simulink library "xpclib"  (Simulink 6.0)
settings: Solver=ode45  SolverMode=SingleTasking  StartTime=0.0  StopTime=10.0  RelTol=1e-3
values from neighbouring files (symbols this model uses):
  base = get_param( gcb, 'base' )    [maddiamondmm.m]    (also in maddiamondmm32frame.m; maddsmm16at.m; mdadsmm16at.m; mdiortddm64x0.m = hex2dec(addr(3:end)))
  block = find_system(bdroot,                          'FollowLinks', 'on',                          'LookUnderMasks', 'all',                          'MaskType', type )    [mdionipci6527.m]
  count = count + 1    (= 5)    [mdecodestate.m]
  port = get_param( gcb, 'port' )    [mdionipci6527.m]    (also in mdiortddm64x0.m = get_param(blocks{i}, 'port'))
undefined symbols (not defined in the file or in its folder): CIO, devid, DIO24, genixlib, get, handlers, irq, mbaseserialmask, mbwaudpmc, mdacbpcidas, mdiamondemeraldmask, mgenix, mmodemcontrol, mquamask, mrs232, msc150checks, mtargetboxleds, mtargetboxwatchdog, mxpccan, PCI, sizeof, vendid
libraries: xpclib x384, simulink x6
(part 3 of 7)

== system xpclib/RS232/Diamond ==
  "Emerald-MM " : Subsystem  PropExecContextAcrossSSBoundary=on
  "Emerald-MM8 " : Subsystem  PropExecContextAcrossSSBoundary=on

== system xpclib/RS232/Mainboard ==
  Baseboard Serial : Subsystem  InitFcn=mbaseserialmask(4,2);  TreatAsAtomicUnit=on  PropExecContextAcrossSSBoundary=on  mask(Baseboard RS232 Send Receive){group=Board Setup, port=1, irqnum=4, saddr1=0x3f8, saddr2=0x3e8, config=Com1/Com3, baud1=115200, parity1=None, ndata1=8, nstop1=1, fifomode1=16 deep, rlevel1=half full, automode1=on, xmtfifosize1=1024, xmtdatatype1=8 bit uint null terminated, rcvfifosize1=1024, rcvmaxread1=1024, rcvminread1=1, rcvusedelim1=on, rcvdelim1=13, rcvdatatype1=count+16 bit uint, rcvsampletime1=-1, baud2=115200, parity2=None, ndata2=8, nstop2=1, fifomode2=16 deep, rlevel2=half full, automode2=off, xmtfifosize2=1024, xmtdatatype2=8 bit uint null terminated, rcvfifosize2=1024, rcvmaxread2=1024, rcvminread2=1, rcvusedelim2=on, rcvdelim2=13, rcvdatatype2=count+16 bit uint, rcvsampletime2=-1}
      mask prompts: group "Parameter group:"; port "Port to modify:"; irqnum "IRQ number:"; saddr1 "First port address:"; saddr2 "Second port address:"; config "Configuration:"; baud1 "Baud rate:"; parity1 "Parity:"; ndata1 "Data bits:"; nstop1 "Stop bits:"; fifomode1 "Hardware fifo size:"; rlevel1 "Receive fifo interrupt level:"; automode1 "Auto RTS/CTS:"; xmtfifosize1 "Transmit software fifo size:"; xmtdatatype1 "Transmit fifo data type:"; rcvfifosize1 "Receive software fifo size:"; rcvmaxread1 "Receive maximum read:"; rcvminread1 "Receive minimum read:"; rcvusedelim1 "Read to delimiter:"; rcvdelim1 "Delimiter:"; rcvdatatype1 "Receive data type:"; rcvsampletime1 "Receive SampleTime:"; baud2 "Baud rate:"; parity2 "Parity:"; ndata2 "Data bits:"; nstop2 "Stop bits:"; fifomode2 "Hardware fifo size:"; rlevel2 "Receive fifo interrupt level:"; automode2 "Auto RTS/CTS:"; xmtfifosize2 "Transmit software fifo size:"; xmtdatatype2 "Transmit fifo data type:"; rcvfifosize2 "Receive software fifo size:"; rcvmaxread2 "Receive maximum read:"; rcvminread2 "Receive minimum read:"; rcvusedelim2 "Read to delimiter:"; rcvdelim2 "Delimiter:"; rcvdatatype2 "Receive data type:"; rcvsampletime2 "Receive SampleTime:"
      mask help:
      | Baseboard
      | RS232 Send Receive Subsystem
      mask init:
      | [addr1, addr2, maskdisplay] = mbaseserialmask( 1, 2 );
      | baddr1 = addr1;
      | baddr2 = addr2;
      | mbaseserialmask( 3, 2 );
      | set_param( gcb, 'MaskDisplay', maskdisplay );
      mask Help: helpview(fullfile(docroot, 'mapfiles', 'xpc.map'), 'Baseboard_Serial_Subsystem')
      mask StyleString: popup(Board Setup|Basic Setup|Transmit Setup|Receive Setup),popup(1|2),edit,edit,edit,popup(Com1/none|Com2/none|Com1/Com3|Com2/Com4|none/Com3|none/Com4|Custom),popup(921600|460800|230400|115200|57600|38400|19200|9600|4800|2400|1200|600|300|110),popup(None|Even|Odd|Mark|Space),popup(5|6|7|8),popup(1|2),popup(64 deep|16 deep|1 deep),popup(1|quarter full|half full|almost full),checkbox,edit,popup(count+32 bit int|count+32 bit uint|count+16 bit int|count+16 bit uint|8 bit int null terminated|8 bit uint null terminated),edit,edit,edit,checkbox,edit,popup(count+32 bit int|count+32 bit uint|count+16 bit int|count+16 bit uint|8 bit int null terminated|8 bit uint null terminated),edit,popup(921600|460800|230400|115200|57600|38400|19200|9600|4800|2400|1200|600|300|110),popup(None|Even|Odd|Mark|Space),popup(5|6|7|8),popup(1|2),popup(64 deep|16 deep|1 deep),popup(1|quarter full|half full|almost full),checkbox,edit,popup(count+32 bit int|count+32 bit uint|count+16 bit int|count+16 bit uint|8 bit int null terminated|8 bit uint null terminated),edit,edit,edit,checkbox,edit,popup(count+32 bit int|count+32 bit uint|count+16 bit int|count+16 bit uint|8 bit int null terminated|8 bit uint null terminated),edit
      mask CallbackString:
      | mbaseserialmask( 2, 2 );
      | |mbaseserialmask( 2, 2 );||||mbaseserialmask( 2, 2 );
      | ||||||||||||||||||||||||||||||||
      mask Display: disp('Baseboard\nRS232\nSend Receive')port_label('input',1,'XMT1');port_label('input',2,'XMT3');port_label('output',1,'RCV1');port_label('output',2,'RCV3');
  Baseboard Serial Internal  blocks : Subsystem  PropExecContextAcrossSSBoundary=on
  Modem Control : S-Function  InitFcn=mmodemcontrol(4)  FunctionName=modemcontrolbase  Parameters=addr, boardtype, rts, dtr, count  mask(Baseboard Modem Control){rts=on, dtr=on, config=Com1, addr=0x3f8}
      mask prompts: config "Configuration:"; addr "Base address:"
      mask help:
      | Baseboard
      | Modem Control
      mask init:
      | count = 0;
      | boardtype = 4;
      | [maskdisplay, count, addr] = mmodemcontrol( 2, rts, dtr, boardtype, config, addr );
      | addr = hex2dec( addr(3:end) );
      | set_param( gcb, 'MaskDisplay', maskdisplay );
      mask Help: helpview(fullfile(docroot, 'mapfiles', 'xpc.map'), 'Baseboard_MODEM_Control')
      mask StyleString: checkbox,checkbox,popup(Com1|Com2|Com3|Com4|Custom),edit
      mask CallbackString:
      | ||mmodemcontrol( 1 );
      | |
      mask Display: disp('Baseboard\nModem Control');port_label('input',1,'RTS');port_label('input',2,'DTR');
  Modem Status : S-Function  FunctionName=modemstatusbase  Parameters=addr, boardtype, cts, dsr, ring, dcd, count, sampletime  mask(Modem Status){cts=on, dsr=on, ring=on, dcd=on, sampletime=-1, config=Com1, addr=0x3f8}
      mask prompts: ring "RI:"; config "Configuration:"; addr "Base address:"
      mask help:
      | Baseboard
      | Modem Status
      mask init:
      | count = 0;
      | boardtype = 4;
      | [maskdisplay, count, addr] = mmodemstatus( 2, cts, dsr, ring, dcd, boardtype, config, addr );
      | addr = hex2dec( addr(3:end) );
      | set_param( gcb, 'MaskDisplay', maskdisplay );
      mask Help: helpview(fullfile(docroot, 'mapfiles', 'xpc.map'), 'Baseboard_MODEM_Status')
      mask StyleString: checkbox,checkbox,checkbox,checkbox,edit,popup(Com1|Com2|Com3|Com4|Custom),edit
      mask CallbackString:
      | |||||mmodemstatus( 1 );
      | |
      mask Display: disp('Baseboard\nModem Status');port_label('output',1,'CTS');port_label('output',2,'DSR');port_label('output',3,'RI');port_label('output',4,'DCD');

== system xpclib/RS232/Quatech ==
  ESC-100 : Subsystem  PropExecContextAcrossSSBoundary=on
  QSC-100 : Subsystem  PropExecContextAcrossSSBoundary=on
  QSC-200/300 : Subsystem  PropExecContextAcrossSSBoundary=on

== system xpclib/RS232/Setup  ==
  S-Function : S-Function  FunctionName=rs232_setup  Parameters=port,baudrate,databit, stopbit, parity, protocol, sendbuf, recbuf, 0

== system xpclib/RS232/Synchronous Mode ==
  note: V1.0 compatible
  "RS232 " : S-Function  FunctionName=rs232sendrec  Parameters=port, inStr, outStr, inport, outport, numinports, numoutports, formatsendinfo, formatrecinfo, waitarg, dtypes, ts, numeom, timeoutarg  mask(rs232sendrec){port=COM1, blockvar=[], ts=0.1}
      mask prompts: blockvar "Message struct name:"; ts "Sample time:"
      mask help:
      | RS-232
      | Mainboard
      | Send/Receive
      mask init:
      | inStr = '';
      | outStr = '';
      | [inStr,outStr,dtypes,maskdisplay,maskdescription,inport,outport, numinports, numoutports, formatsendinfo, formatrecinfo, waitarg, numeom, timeoutarg] = mrs232 (1, blockvar, 3);
      | set_param(gcb,'MaskDisplay',maskdisplay);
      | set_param(gcb,'MaskDescription',maskdescription);
      mask Help: helpview(fullfile(docroot, 'mapfiles', 'xpc.map'), 'RS232_Synchronous-Mode_RS232')
      mask StyleString: popup(COM1|COM2|COM3|COM4),edit,edit
      mask Display: disp('RS-232\nMainboard\nSend/Receive');
  "Send & Receive " : Subsystem  PropExecContextAcrossSSBoundary=on  mask(rs232sendrec){port=COM2, formatsend='start,%f,stop;', formatrec='start,%f,stop;', numb=1, ts=0.01}
      mask prompts: formatsend "Send format:"; formatrec "Receive format:"; numb "Number of end-of-message characters:"; ts "Sample time:"
      mask Help: helpview(fullfile(docroot, 'mapfiles', 'xpc.map'), 'RS232_Synchronous-Mode_Send-&-Receive')
      mask StyleString: popup(COM1|COM2|COM3|COM4),edit,edit,edit,edit
      mask Display: disp('RS232\nMainboard\nSend/Receive');

== system xpclib/Shared Memory/SBS Broadcast Memory ==
  "SBS25x0 init " : S-Function  FunctionName=memsbs25x0init  Parameters=get(node,'BT_REG_CTRL_ARG'),get(node,'BT_REG_MEM_ARG'),get(node,'WIT'),[],pci  mask(SBS 25x0 Initialization){node=[], pci=-1}
      mask prompts: node "Node struct:"; pci "PCI slot (-1: autosearch)"
      mask help: Configures 5565 shared-memory board produced by VMIC Inc. This is a required block for any model that uses shared memory with the VMIC 5565. It configures important registers on the board according to the user-defined node structure.
      mask init:
      | node=smnodesbs25x0(node);
      mask Help: helpview(fullfile(docroot, 'mapfiles', 'xpc.map'),'SBS_25x0_Init')
      mask Display: disp('init')
  "SBS25x0 read " : S-Function  FunctionName=memsbs25x0read  Parameters=base(partition(1)), sizeof(partition(1)),ts, pci, errport  mask(SBS 25x0 Read){partition=[], ts=0.001, pci=-1, errport=off}
      mask prompts: partition "Partition struct:"; ts "Sampletime:"; pci "PCI slot (-1: autosearch)"; errport "Error Status Port"
      mask help: Reads blocks of data (32-bit words) from shared memory. Should be combined with '5565 unpack' to define data partitioning.
      mask init:
      | partition=smpartsbs25x0(partition);
      mask Help: helpview(fullfile(docroot, 'mapfiles', 'xpc.map'),'SBS_25x0_Read')
      mask Display:
      | disp('read')
      | port_label('output',1,'ud')
  "SBS25x0 write " : S-Function  FunctionName=memsbs25x0write  Parameters=base(partition(1)), sizeof(partition(1)),ts, pci, errport  mask(SBS 25x0 Write){partition=[], ts=0.001, pci=-1, errport=off}
      mask prompts: partition "Partition struct:"; ts "Sampletime:"; pci "PCI slot (-1: autosearch)"; errport "Error Status Port"
      mask help: Writes blocks of data (32-bit words) to shared-memory. Should be combined with '5565 pack' to define data partitioning.
      mask init:
      | partition=smpartsbs25x0(partition);
      mask Help: helpview(fullfile(docroot, 'mapfiles', 'xpc.map'),'SBS_25x0_Write')
      mask Display: disp('write')

== system xpclib/Shared Memory/Systran ==
  Change endianess : xpclib/Shared Memory/Change endianess  numInp=1  lengthIn=Byte
  "SC150 init " : S-Function  InitFcn=msc150checks(1)  FunctionName=memscramnetinit  Parameters=node.Interface.Internal.CSRs, node.Interface.Internal.ACRAMinfo, pci  mask(SC150 Init){node=[], pci=-1}
      mask prompts: node "Node struct:"; pci "PCI slot (-1: autosearch)"
      mask help:
      | SC150
      | Systran
      | Initialization
      mask init:
      | node=completenodestruct(node);
      mask Help: helpview(fullfile(docroot, 'mapfiles', 'xpc.map'),'Systran_SC150_Init')
      mask Display: disp('init')
  "SC150 pack " : xpclib/Shared Memory/Shared Memory Pack   partition=[]
  "SC150 read " : S-Function  FunctionName=memscramnetread  Parameters=partition(1).Internal.Address, partition(1).Internal.NDwords, ts, pci  mask(SC150 Read){partition=[], ts=0.001, pci=-1}
      mask prompts: partition "Partition struct:"; ts "Sampletime:"; pci "PCI slot (-1: autosearch)"
      mask help:
      | SC150
      | Systran
      | Read
      mask init:
      | partition=completepartitionstruct(partition);
      mask Help: helpview(fullfile(docroot, 'mapfiles', 'xpc.map'),'Systran_SC150_Read')
      mask Display: disp('read')
  SC150 rearm : S-Function  FunctionName=memscramnetrearm  Parameters=partition.Internal.Address, partition.Internal.NDwords, ts, pci  mask(SC150 Rearm){partition=[], ts=0.001, pci=-1}
      mask prompts: partition "Partition struct:"; ts "Sampletime:"; pci "PCI slot (-1: autosearch)"
      mask help:
      | SC150
      | Systran
      | Rearm
      mask init:
      | partition=completepartitionstruct(partition);
      mask Help: helpview(fullfile(docroot, 'mapfiles', 'xpc.map'),'Systran_SC150_Rearm')
      mask Display: disp('rearm')
  "SC150 unpack " : xpclib/Shared Memory/Shared Memory Unpack   partition=[]
  "SC150 write " : S-Function  FunctionName=memscramnetwrite  Parameters=partition(1).Internal.Address, partition(1).Internal.NDwords, ts, pci  mask(SC150 Write){partition=[], ts=0.001, pci=-1}
      mask prompts: partition "Partition struct:"; ts "Sampletime:"; pci "PCI slot (-1: autosearch)"
      mask help:
      | SC150
      | Systran
      | Write
      mask init:
      | partition=completepartitionstruct(partition);
      mask Help: helpview(fullfile(docroot, 'mapfiles', 'xpc.map'),'Systran_SC150_Write')
      mask Display: disp('write')

== system xpclib/Shared Memory/VMIC ==
  5565 broadcast : S-Function  FunctionName=mem5565netbroadcast  Parameters=ninterrupt,target, ts, pci  mask(5565 Network Interrupts){target=-1, ninterrupt=1, ts=0.001, pci=-1}
      mask prompts: target "Target Node (-1 : Global)"; ninterrupt "Interrupt Number"; ts "Sampletime:"; pci "PCI slot (-1: autosearch)"
      mask help: Generates network interrupts at the specified sample rate.
      mask Help: helpview(fullfile(docroot, 'mapfiles', 'xpc.map'),'VMIC_5565_Broadcast')
      mask StyleString: edit,popup(1|2|3|Initialization),edit,edit
      mask Display:
      | disp('Broadcast')
      | port_label('Input',1,'En')
      | port_label('Input',2,'Data')
  "5565 init " : S-Function  FunctionName=mem5565netinit  Parameters=node.Interface.Internal.LCSR1, node.Interface.Internal.LIER,node.Interface.Internal.INodeID,pci  mask(5565 Initialization){node=[], pci=-1}
      mask prompts: node "Node struct:"; pci "PCI slot (-1: autosearch)"
      mask help: Configures 5565 shared-memory board produced by VMIC Inc. This is a required block for any model that uses shared memory with the VMIC 5565. It configures important registers on the board according to the user-defined node structure.
      mask init:
      | node=completenodestruct(node,'5565');
      mask Help: helpview(fullfile(docroot, 'mapfiles', 'xpc.map'),'VMIC_5565_Init')
      mask Display: disp('init')
  "5565 pack " : xpclib/Shared Memory/Shared Memory Pack   partition=[]
  "5565 read " : S-Function  FunctionName=mem5565netread  Parameters=partition(1).Internal.Address, partition(1).Internal.NDwords, ts, pci, errport  mask(5565 Memory Read){partition=[], ts=0.001, pci=-1, errport=off}
      mask prompts: partition "Partition struct:"; ts "Sampletime:"; pci "PCI slot (-1: autosearch)"; errport "Error Status Port"
      mask help: Reads blocks of data (32-bit words) from shared memory. Should be combined with '5565 unpack' to define data partitioning.
      mask init:
      | partition=completepartitionstruct(partition);
      mask Help: helpview(fullfile(docroot, 'mapfiles', 'xpc.map'),'VMIC_5565_Read')
      mask Display:
      | disp('read')
      | port_label('output',1,'ud')
  "5565 unpack  " : xpclib/Shared Memory/Shared Memory Unpack   partition=[]
  "5565 write " : S-Function  FunctionName=mem5565netwrite  Parameters=partition(1).Internal.Address, partition(1).Internal.NDwords, ts, pci, errport  mask(5565 Write){partition=[], ts=0.001, pci=-1, errport=off}
      mask prompts: partition "Partition struct:"; ts "Sampletime:"; pci "PCI slot (-1: autosearch)"; errport "Error Status Port"
      mask help: Writes blocks of data (32-bit words) to shared-memory. Should be combined with '5565 pack' to define data partitioning.
      mask init:
      | partition=completepartitionstruct(partition);
      mask Help: helpview(fullfile(docroot, 'mapfiles', 'xpc.map'),'VMIC_5565_Write')
      mask Display: disp('write')
  Change endianess : xpclib/Shared Memory/Change endianess  numInp=1  lengthIn=Byte

== system xpclib/Signal Conditioning/add2 ==
  "CIO-DIO24 " : S-Function  AncestorBlock=genixlib/CIO-DIO24  LoadFcn=mgenix(1)  InitFcn=mgenix(1)  FunctionName=genixisa8255  Parameters=initData, offset8255, baseAddress, control8255  mask(genixisa8255){fileName=, baseaddress=0x300}
      mask prompts: fileName "Genix initialization file (path\file):"; baseaddress "Base address (i.e. 0xd000):"
      mask help:
      | CIO-DIO24
      | ComputerBoards
      | Genix
      mask init:
      | baseAddress=hex2dec(baseaddress(3:end));
      | boardType=1;
      | control8255=0;
      | offset8255=0;
      | initData=[];
      | [initData, offset8255, control8255]=mgenix(2, fileName, baseAddress, 1);
      mask Help: helpview(fullfile(docroot, 'mapfiles', 'xpc.map'), 'add2_CIO-DIO24_SignalConditioning')
      mask Display: disp('CIO-DIO24\nComputerBoards\nGenix');
  "PCI-DIO24 " : S-Function  AncestorBlock=genixlib/PCI-DIO24  LoadFcn=mgenix(1)  InitFcn=mgenix(1)  FunctionName=genixpci8255  Parameters=initData, offset8255, pciSlot, control8255  mask(genixpci8255){fileName=, pciSlot=-1}
      mask prompts: fileName "Genix initialization file (path\file):"; pciSlot "PCI slot (-1: autosearch):"
      mask help:
      | PCI-DIO24
      | ComputerBoards
      | Genix
      mask init:
      | boardType=1;
      | control8255=0;
      | offset8255=0;
      | initData=[];
      | [initData, offset8255, control8255]=mgenix(2, fileName, pciSlot, 2);
      mask Help: helpview(fullfile(docroot, 'mapfiles', 'xpc.map'), 'add2_PCI-DIO24_SignalConditioning')
      mask Display: disp('PCI-DIO24\nComputerBoards\nGenix');

== system xpclib/Synchro Resolver/NAII ==

== system xpclib/Synchro Resolver/SBS  Technologies ==

== system xpclib/Thermo couple/Measurement Computing ==

== system xpclib/Watchdog/Acces IO ==
  "WDG-CSM " : S-Function  FunctionName=wdaciowdgcsm  Parameters=wdtime,showreset,sampletime,baseaddress  mask(wdaciowdgcsm){wdtime=1, showreset=off, sampletime=0.001, baseaddress=0x300}
      mask prompts: wdtime "Watchdog time [s] (20us-4800s):"; showreset "Show reset port"; sampletime "Sample time:"; baseaddress "Base address (i.e. 0xd000):"
      mask help:
      | WDG-CSM
      | ACCES I/O
      | Watchdog
      mask init:
      | baseaddress=hex2dec(baseaddress(3:end));
      mask Help: helpview(fullfile(docroot, 'mapfiles', 'xpc.map'), 'AccesIO_WDG-CSM_Watchdog')
      mask Display: disp('WDG-CSM\nACCES I/O\nWatchdog');

== system xpclib/Watchdog/MathWorks ==
  Watchdog : S-Function  InitFcn=mtargetboxwatchdog(1);  FunctionName=targetboxwatchdog  Parameters=units, interval, portReset, kybdReset, mouseReset, reboot, sampleTime  mask(targetboxwatchdog){units=seconds, interval=255, portReset=on, kybdReset=off, mouseReset=off, reboot=off, sampleTime=0.001}
      mask prompts: units "Timeout units:"; interval "Timeout interval (1-255):"; portReset "Show reset port (R)"; kybdReset "Reset upon keyboard activity"; mouseReset "Reset upon mouse activity"; reboot "Reboot upon expiration of watchdog"; sampleTime "Sample time:"
      mask help:
      | TargetBox 10x120x
      | The MathWorks
      | Watchdog
      mask init:
      | phase = 2;
      | [maskDisplay, maskDescription] = mtargetboxwatchdog( phase, interval, portReset, sampleTime );
      | set_param(gcb,'MaskDescription',maskDescription);
      | set_param(gcb,'MaskDisplay',maskDisplay);
      mask Help: helpview(fullfile(docroot, 'mapfiles', 'xpc_targetbox.map'), 'TheMathWorks_TargetBox10x120x_Watchdog')
      mask StyleString: popup(seconds|minutes),edit,checkbox,checkbox,checkbox,checkbox,edit
      mask Display: disp('TargetBox 10x120x\nThe MathWorks\nWatchdog');port_label('input', 1, 'R');

== system xpclib/Watchdog/Versalogic ==

== system xpclib/CAN/Softing/CAN-AC2-104 SJA 1000 ==
  FIFO Mode : Subsystem  PropExecContextAcrossSSBoundary=on
  "Receive " : S-Function  FunctionName=canac2104receive  Parameters=canPort, ids, ididx, output, ts, board  mask(canac2104receive){board=1, canPort=CAN 1, range=Standard (11-bit), ids=[0], output=Data, inten=off, ts=0.001, ididx=[0]}
      mask prompts: canPort "CAN port:"; range "CAN identifier range:"; ids "Identifiers:"; output "Output port options:"; inten "Generate interrupts"; ts "Sample time:"
      mask help:
      | Softing
      | CAN-AC2-104
      | with SJA1000
      mask init:
      | mxpccanicon('CAN-AC2-104','Receive',canPort,range,ids,board)
      mask Help: helpview(fullfile(docroot, 'mapfiles', 'xpc.map'), 'Softing_CAN-AC2-104-SJA-1000_Receive')
      mask StyleString: popup(1|2|3),popup(CAN 1|CAN 2),popup(Standard (11-bit)|Extended (29-bit)),edit,popup(Data|Data - Status|Data - Timestamp|Data - Status - Timestamp),checkbox,edit,edit
      mask Display: text(0.05,0.75,'CAN-AC2-104 B1','horizontalAlignment','left');text(0.05,0.5,'CAN 1 - Receive','horizontalAlignment','left');text(0.05,0.25,'Standard 11bit','horizontalAlignment','left');port_label('output',1,'0');
  "Send " : S-Function  FunctionName=canac2104send  Parameters=canPort, ids, ididx, output, ts, sizesout, board  mask(canac2104send){board=1, canPort=CAN 1, range=Standard (11-bit), ids=[0], sizes=[8], output=off, ts=0.001, ididx=[0]}
      mask prompts: canPort "CAN port:"; range "CAN identifier range:"; ids "Identifiers:"; sizes "Data frame sizes:"; output "Show status output ports"; ts "Sample time:"
      mask help:
      | Softing
      | CAN-AC2-104
      | with SJA1000
      mask init:
      | if isempty(sizes), sizesout=8; end;
      | if length(sizes)==1, sizesout=sizes*ones(1,length(ids)); else, sizesout=sizes; end;
      | if length(sizesout)~=length(ids), error('Identifier vector and Data Frame Size Vector must have the same length');end
      | if ~isempty(find(sizesout<1|sizesout>8)), error('Data Frame Sizes must be in the range 1..8'); end;
      | mxpccanicon('CAN-AC2-104','Send',canPort,range,ids,board)
      mask Help: helpview(fullfile(docroot, 'mapfiles', 'xpc.map'), 'Softing_CAN-AC2-104-SJA-1000_Send')
      mask StyleString: popup(1|2|3),popup(CAN 1|CAN 2),popup(Standard (11-bit)|Extended (29-bit)),edit,edit,checkbox,edit,edit
      mask Display: text(0.98,0.75,'CAN-AC2-104 B1','horizontalAlignment','right');text(0.98,0.5,'CAN 1 - Send','horizontalAlignment','right');text(0.98,0.25,'Standard 11bit','horizontalAlignment','right');port_label('input',1,'0');
  "Setup " : S-Function  InitFcn=mxpccan(1);  FunctionName=canac2104setup  Parameters=can1UserBR, can2UserBR, can1SendS, can1RecS, can2SendS, can2RecS, can1SendE, can1RecE, can2SendE, can2RecE, can1RecSI, can1RecEI, can2RecSI, can2RecEI, initarray, termarray, ioBaseAddress, memBaseAddress, intNo, board  mask(canac2104setup){board=1, can1Baudrate=1 MBaud, can1UserBR=[1,1,4,3], can2Baudrate=1 MBaud, can2UserBR=[1,1,4,3], init=[], term=[], ioBaseAddressL=0x300, memBaseAddressL=0xd0000, intNo=None}
      mask prompts: can1Baudrate "CAN 1 - baud rate:"; can1UserBR "CAN 1 - user defined baud rate:"; can2Baudrate "CAN 2 - baud rate:"; can2UserBR "CAN 2 - user defined baud rate:"; init "Initialization command structure:"; term "Termination:"; ioBaseAddressL "I/O base address:"; memBaseAddressL "Memory base address:"; intNo "Interrupt line:"
      mask help:
      | Softing
      | CAN-AC2-104
      | with SJA1000
      mask init:
      | initarray=0;
      | termarray=0;
      | ioBaseAddress=768;
      | memBaseAddress=819200;
      | if strcmp(intNo,'None'), intNo='0'; end
      | intNo=str2num(intNo);
      | [can1UserBR, can2UserBR, can1SendS, can1SendE, can2SendS, can2SendE, can1RecS, can1RecE, can2RecS, can2RecE, can1RecSI, can1RecEI, can2RecSI, can2RecEI, initarray, termarray, ioBaseAddress, memBaseAddress]= mxpccan(2, 1, can1Baudrate, can1UserBR, can2Baudrate, can2UserBR, init, term, ioBaseAddressL, memBaseAddressL, board);
      mask Help: helpview(fullfile(docroot, 'mapfiles', 'xpc.map'), 'Softing_CAN-AC2-104-SJA-1000_Setup')
      mask StyleString: popup(1|2|3),popup(1 MBaud|800 kBaud|500 kBaud|250 kBaud|125 kBaud|100 kBaud|10 kBaud|User defined),edit,popup(1 MBaud|800 kBaud|500 kBaud|250 kBaud|125 kBaud|100 kBaud|10 kBaud|User defined),edit,edit,edit,edit,edit,popup(None|5|9|10|11|12|15)
      mask Display: disp(['CAN-AC2-104 B',num2str(board),'\nCAN 1 / CAN 2\nStandard / Extended'])

== system xpclib/CAN/Softing/CAN-AC2-ISA Intel 527 ==
  "Receive " : S-Function  FunctionName=canac2isaereceive  Parameters=canPort, ids, ididx, output, ts, board  mask(canac2isaereceive){board=1, canPort=CAN 1, range=Standard (11-bit), ids=[0], output=Data, inten=off, ts=0.001, ididx=[0]}
      mask prompts: canPort "CAN port:"; range "CAN identifier range:"; ids "Identifiers:"; output "Output port options:"; inten "Generate interrupts"; ts "Sample time:"
      mask help:
      | Softing
      | CAN-AC2-ISA
      | with Intel 82527
      mask init:
      | board=0;
      | mxpccanicon('CAN-AC2-ISA','Receive',canPort,range,ids,board)
      mask Help: helpview(fullfile(docroot, 'mapfiles', 'xpc.map'), 'Softing_CAN-AC2-ISA-Intel-527_Receive')
      mask StyleString: popup(1|2|3),popup(CAN 1|CAN 2),popup(Standard (11-bit)|Extended (29-bit)),edit,popup(Data|Data - Status|Data - Timestamp|Data - Status - Timestamp),checkbox,edit,edit
      mask Display: text(0.05,0.75,'CAN-AC2-ISA','horizontalAlignment','left');text(0.05,0.5,'CAN 1 - Receive','horizontalAlignment','left');text(0.05,0.25,'Standard 11bit','horizontalAlignment','left');port_label('output',1,'0');
  "Send " : S-Function  FunctionName=canac2isaesend  Parameters=canPort, ids, ididx, output, ts, sizesout, board  mask(canac2isaesend){board=1, canPort=CAN 1, range=Standard (11-bit), ids=[0], sizes=[8], output=off, ts=0.001, ididx=[0]}
      mask prompts: canPort "CAN port:"; range "CAN identifier range:"; ids "Identifiers:"; sizes "Data frame sizes:"; output "Show status output ports"; ts "Sample time:"
      mask help:
      | Softing
      | CAN-AC2-ISA
      | with Intel 82527
      mask init:
      | if isempty(sizes), sizesout=8; end;
      | if length(sizes)==1, sizesout=sizes*ones(1,length(ids)); else, sizesout=sizes; end;
      | if length(sizesout)~=length(ids), error('Identifier vector and Data Frame Size Vector must have the same length');end
      | if ~isempty(find(sizesout<1|sizesout>8)), error('Data Frame Sizes must be in the range 1..8'); end;
      | board=0;
      | mxpccanicon('CAN-AC2-ISA','Send',canPort,range,ids,board)
      mask Help: helpview(fullfile(docroot, 'mapfiles', 'xpc.map'), 'Softing_CAN-AC2-ISA-Intel-527_Send')
      mask StyleString: popup(1|2|3),popup(CAN 1|CAN 2),popup(Standard (11-bit)|Extended (29-bit)),edit,edit,checkbox,edit,edit
      mask Display: text(0.98,0.75,'CAN-AC2-ISA','horizontalAlignment','right');text(0.98,0.5,'CAN 1 - Send','horizontalAlignment','right');text(0.98,0.25,'Standard 11bit','horizontalAlignment','right');port_label('input',1,'0');
  "Setup " : S-Function  InitFcn=mxpccan(1);  FunctionName=canac2isaesetup  Parameters=can1UserBR, can2UserBR, can1SendS, can1RecS, can2SendS, can2RecS, can1SendE, can1RecE, can2SendE, can2RecE, can1RecSI, can1RecEI, can2RecSI, can2RecEI, initarray, termarray, ioBaseAddress, memBaseAddress, intNo, board  mask(canac2isaesetup){board=1, can1Baudrate=1 MBaud, can1UserBR=[1,1,4,3], can2Baudrate=1 MBaud, can2UserBR=[1,1,4,3], init=[], term=[], memBaseAddressL=2 (16k): D4000-D7FFF}
      mask prompts: can1Baudrate "CAN 1 - baud rate:"; can1UserBR "CAN 1 - user defined baud rate:"; can2Baudrate "CAN 2 - baud rate:"; can2UserBR "CAN 2 - user defined baud rate:"; init "Initialization command structure:"; term "Termination:"; memBaseAddressL "Memory base address (i.e. 0xd000):"
      mask help:
      | Softing
      | CAN-AC2-ISA
      | with Intel 82527
      mask init:
      | board=1;
      | initarray=0;
      | termarray=0;
      | ioBaseAddress=768;
      | ioBaseAddressL='0x300';
      | memBaseAddress=819200;
      | intNo='None';
      | if strcmp(intNo,'None'), intNo='0'; end
      | intNo=str2num(intNo);
      | [can1UserBR, can2UserBR, can1SendS, can1SendE, can2SendS, can2SendE, can1RecS, can1RecE, can2RecS, can2RecE, can1RecSI, can1RecEI, can2RecSI, can2RecEI, initarray, termarray, ioBaseAddress, memBaseAddress]= mxpccan(2, 4, can1Baudrate, can1UserBR, can2Baudrate, can2UserBR, init, term, ioBaseAddressL, memBaseAddressL, board);
      | ioBaseAddress=768;
      | memBaseAddress=memBaseAddressL;
      mask Help: helpview(fullfile(docroot, 'mapfiles', 'xpc.map'), 'Softing_CAN-AC2-ISA-Intel-527_Setup')
      mask StyleString: popup(1),popup(1 MBaud|800 kBaud|500 kBaud|250 kBaud|125 kBaud|100 kBaud|10 kBaud|User defined),edit,popup(1 MBaud|800 kBaud|500 kBaud|250 kBaud|125 kBaud|100 kBaud|10 kBaud|User defined),edit,edit,edit,popup(0 (64k): D0000-DFFFF|1 (16k): D0000-D3FFF|2 (16k): D4000-D7FFF|3 (16k): D8000-D8FFF|4 (16k): DC000-DFFFF|5 (16k): E0000-E3FFF|6 (16k): E4000-E7FFF|7 (64k): E0000-EFFFF)
      mask Display: disp(['CAN-AC2-ISA E','\nCAN 1 / CAN 2\nStandard / Extended'])

== system xpclib/CAN/Softing/CAN-AC2-ISA Philips C200 ==
  "Receive " : S-Function  FunctionName=canac2isareceive  Parameters=canPort, ids, ididx, output, ts, board  mask(canac2isareceive){board=1, canPort=CAN 1, range=Standard (11-bit), ids=[0], output=Data, inten=off, ts=0.001, ididx=[0]}
      mask prompts: canPort "CAN port:"; range "CAN identifier range:"; ids "Identifiers:"; output "Output port options:"; inten "Generate interrupts"; ts "Sample time:"
      mask help:
      | Softing
      | CAN-AC2-ISA
      | with Philips PCA 82C200
      mask init:
      | board=0;
      | mxpccanicon('CAN-AC2-ISA','Receive',canPort,range,ids,board)
      mask Help: helpview(fullfile(docroot, 'mapfiles', 'xpc.map'), 'Softing_CAN-AC2-ISA-Philips-C200_Receive')
      mask StyleString: popup(1|2|3),popup(CAN 1|CAN 2),popup(Standard (11-bit)|Extended (29-bit)),edit,popup(Data|Data - Status|Data - Timestamp|Data - Status - Timestamp),checkbox,edit,edit
      mask Display: text(0.05,0.75,'CAN-AC2-ISA','horizontalAlignment','left');text(0.05,0.5,'CAN 1 - Receive','horizontalAlignment','left');text(0.05,0.25,'Standard 11bit','horizontalAlignment','left');port_label('output',1,'0');
  "Send " : S-Function  FunctionName=canac2isasend  Parameters=canPort, ids, ididx, output, ts, sizesout, board  mask(canac2isasend){board=1, canPort=CAN 1, range=Standard (11-bit), ids=[0], sizes=[8], output=off, ts=0.001, ididx=[0]}
      mask prompts: canPort "CAN port:"; range "CAN identifier range:"; ids "Identifiers:"; sizes "Data frame sizes:"; output "Show status output ports"; ts "Sample time:"
      mask help:
      | Softing
      | CAN-AC2-ISA
      | with Philips PCA 82C200
      mask init: same as xpclib/CAN/Softing/CAN-AC2-ISA Intel 527/Send 
      mask Help: helpview(fullfile(docroot, 'mapfiles', 'xpc.map'), 'Softing_CAN-AC2-ISA-Philips-C200_Send')
      mask StyleString: popup(1|2|3),popup(CAN 1|CAN 2),popup(Standard (11-bit)|Extended (29-bit)),edit,edit,checkbox,edit,edit
      mask Display: text(0.98,0.75,'CAN-AC2-ISA','horizontalAlignment','right');text(0.98,0.5,'CAN 1 - Send','horizontalAlignment','right');text(0.98,0.25,'Standard 11bit','horizontalAlignment','right');port_label('input',1,'0');
  "Setup " : S-Function  InitFcn=mxpccan(1);  FunctionName=canac2isasetup  Parameters=can1UserBR, can2UserBR, can1SendS, can1RecS, can2SendS, can2RecS, can1SendE, can1RecE, can2SendE, can2RecE, can1RecSI, can1RecEI, can2RecSI, can2RecEI, initarray, termarray, ioBaseAddress, memBaseAddress, intNo, board  mask(canac2isasetup){board=1, can1Baudrate=1 MBaud, can1UserBR=[1,1,4,3], can2Baudrate=1 MBaud, can2UserBR=[1,1,4,3], init=[], term=[], memBaseAddressL=2 (16k): D4000-D7FFF}
      mask prompts: can1Baudrate "CAN 1 - baud rate:"; can1UserBR "CAN 1 - user defined baud rate:"; can2Baudrate "CAN 2 - baud rate:"; can2UserBR "CAN 2 - user defined baud rate:"; init "Initialization command structure:"; term "Termination:"; memBaseAddressL "Memory base address (i.e. 0xd000):"
      mask help:
      | Softing
      | CAN-AC2-ISA
      | with Philips PCA 82C200
      mask init:
      | board=1;
      | initarray=0;
      | termarray=0;
      | ioBaseAddress=768;
      | ioBaseAddressL='0x300';
      | memBaseAddress=819200;
      | intNo='None';
      | if strcmp(intNo,'None'), intNo='0'; end
      | intNo=str2num(intNo);
      | [can1UserBR, can2UserBR, can1SendS, can1SendE, can2SendS, can2SendE, can1RecS, can1RecE, can2RecS, can2RecE, can1RecSI, can1RecEI, can2RecSI, can2RecEI, initarray, termarray, ioBaseAddress, memBaseAddress]= mxpccan(2, 3, can1Baudrate, can1UserBR, can2Baudrate, can2UserBR, init, term, ioBaseAddressL, memBaseAddressL, board);
      | ioBaseAddress=768;
      | memBaseAddress=memBaseAddressL;
      mask Help: helpview(fullfile(docroot, 'mapfiles', 'xpc.map'), 'Softing_CAN-AC2-ISA-Philips-C200_Setup')
      mask StyleString: popup(1),popup(1 MBaud|800 kBaud|500 kBaud|250 kBaud|125 kBaud|100 kBaud|10 kBaud|User defined),edit,popup(1 MBaud|800 kBaud|500 kBaud|250 kBaud|125 kBaud|100 kBaud|10 kBaud|User defined),edit,edit,edit,popup(0 (64k): D0000-DFFFF|1 (16k): D0000-D3FFF|2 (16k): D4000-D7FFF|3 (16k): D8000-D8FFF|4 (16k): DC000-DFFFF|5 (16k): E0000-E3FFF|6 (16k): E4000-E7FFF|7 (64k): E0000-EFFFF)
      mask Display: disp(['CAN-AC2-ISA ','\nCAN 1 / CAN 2\nStandard'])

== system xpclib/CAN/Softing/CAN-AC2-PCI SJA 1000 ==
  FIFO Mode : Subsystem  PropExecContextAcrossSSBoundary=on
  "Receive " : S-Function  FunctionName=canac2pcireceive  Parameters=canPort, ids, ididx, output, ts, board  mask(canac2pcireceive){board=1, canPort=CAN 1, range=Standard (11-bit), ids=[0], output=Data, inten=off, ts=0.001, ididx=[0]}
      mask prompts: canPort "CAN port:"; range "CAN identifier range:"; ids "Identifiers:"; output "Output port options:"; inten "Generate interrupts"; ts "Sample time:"
      mask help:
      | Softing
      | CAN-AC2-PCI
      | with SJA1000
      mask init:
      | mxpccanicon('CAN-AC2-PCI','Receive',canPort,range,ids,board)
      mask Help: helpview(fullfile(docroot, 'mapfiles', 'xpc.map'), 'Softing_CAN-AC2-PCI-SJA-1000_Receive')
      mask StyleString: popup(1|2|3),popup(CAN 1|CAN 2),popup(Standard (11-bit)|Extended (29-bit)),edit,popup(Data|Data - Status|Data - Timestamp|Data - Status - Timestamp),checkbox,edit,edit
      mask Display: text(0.05,0.75,'CAN-AC2-PCI B1','horizontalAlignment','left');text(0.05,0.5,'CAN 1 - Receive','horizontalAlignment','left');text(0.05,0.25,'Standard 11bit','horizontalAlignment','left');port_label('output',1,'0');
  "Send " : S-Function  FunctionName=canac2pcisend  Parameters=canPort, ids, ididx, output, ts, sizesout, board  mask(canac2pcisend){board=1, canPort=CAN 1, range=Standard (11-bit), ids=[0], sizes=[8], output=off, ts=0.001, ididx=[0]}
      mask prompts: canPort "CAN port:"; range "CAN identifier range:"; ids "Identifiers:"; sizes "Data frame sizes:"; output "Show status output ports"; ts "Sample time:"
      mask help:
      | Softing
      | CAN-AC2-PCI
      | with SJA1000
      mask init:
      | if isempty(sizes), sizesout=8; end;
      | if length(sizes)==1, sizesout=sizes*ones(1,length(ids)); else, sizesout=sizes; end;
      | if length(sizesout)~=length(ids), error('Identifier vector and Data Frame Size Vector must have the same length');end
      | if ~isempty(find(sizesout<1|sizesout>8)), error('Data Frame Sizes must be in the range 1..8'); end;
      | mxpccanicon('CAN-AC2-PCI','Send',canPort,range,ids,board)
      mask Help: helpview(fullfile(docroot, 'mapfiles', 'xpc.map'), 'Softing_CAN-AC2-PCI-SJA-1000_Send')
      mask StyleString: popup(1|2|3),popup(CAN 1|CAN 2),popup(Standard (11-bit)|Extended (29-bit)),edit,edit,checkbox,edit,edit
      mask Display: text(0.98,0.75,'CAN-AC2-PCI B1','horizontalAlignment','right');text(0.98,0.5,'CAN 1 - Send','horizontalAlignment','right');text(0.98,0.25,'Standard 11bit','horizontalAlignment','right');port_label('input',1,'0');
  "Setup " : S-Function  InitFcn=mxpccan(1);  FunctionName=canac2pcisetup  Parameters=can1UserBR, can2UserBR, can1SendS, can1RecS, can2SendS, can2RecS, can1SendE, can1RecE, can2SendE, can2RecE, can1RecSI, can1RecEI, can2RecSI, can2RecEI, initarray, termarray, ioBaseAddress, memBaseAddress, intNo, board, can1bus, can2bus  mask(canac2pcisetup){board=1, can1bus=Highspeed (ISO 11898), can1Baudrate=1 MBaud, can1UserBR=[1,1,4,3], can2bus=Highspeed (ISO 11898), can2Baudrate=1 MBaud, can2UserBR=[1,1,4,3], init=[], term=[], ioBaseAddress=-1}
      mask prompts: can1bus "CAN 1 - physical bus:"; can1Baudrate "CAN 1 - baud rate:"; can1UserBR "CAN 1 - user defined baud rate:"; can2bus "CAN 2 - physical bus:"; can2Baudrate "CAN 2 - baud rate:"; can2UserBR "CAN 2 - user defined baud rate:"; init "Initialization command structure:"; term "Termination:"; ioBaseAddress "PCI slot (-1: autosearch):"
      mask help:
      | Softing
      | CAN-AC2-PCI
      | with SJA1000
      mask init:
      | can1str='';can2str='';
      | if can1bus==2, can1str=' LS'; end;if can2bus==2, can2str=' LS'; end;
      | initarray=0;
      | termarray=0;
      | ioBaseAddressL='0'; memBaseAddressL='0';
      | memBaseAddress=819200;
      | intNo=0;
      | [can1UserBR, can2UserBR, can1SendS, can1SendE, can2SendS, can2SendE, can1RecS, can1RecE, can2RecS, can2RecE, can1RecSI, can1RecEI, can2RecSI, can2RecEI, initarray, termarray]= mxpccan(2, 2, can1Baudrate, can1UserBR, can2Baudrate, can2UserBR, init, term, ioBaseAddressL, memBaseAddressL, board);
      mask Help: helpview(fullfile(docroot, 'mapfiles', 'xpc.map'), 'Softing_CAN-AC2-PCI-SJA-1000_Setup')
      mask StyleString: popup(1|2|3),popup(Highspeed (ISO 11898) |Lowspeed (requires LS module)),popup(1 MBaud|800 kBaud|500 kBaud|250 kBaud|125 kBaud|100 kBaud|10 kBaud|User defined),edit,popup(Highspeed (ISO 11898) |Lowspeed (requires LS module)),popup(1 MBaud|800 kBaud|500 kBaud|250 kBaud|125 kBaud|100 kBaud|10 kBaud|User defined),edit,edit,edit,edit
      mask Display: disp(['CAN-AC2-PCI B',num2str(board),'\nCAN 1',can1str,' / CAN 2',can2str,'\nStandard / Extended'])

== system xpclib/CAN/Utilities/CAN Timeout Detection ==
  u : Inport  LatchInput=off
  Fcn : Fcn  Expr=u>timeout
  Gain1 : Gain  Gain=-1  SaturateOnIntegerOverflow=on
  Memory : Memory  InheritSampleTime=on
  Probe : Probe  ProbeWidth=off  ProbeComplexSignal=off  ProbeSignalDimensions=on
  Relational Operator : RelationalOperator  Operator===  InputSameDT=on
  Sum : Sum  SaturateOnIntegerOverflow=on  InputSameDT=on
  Switch : Switch  Orientation=left  Threshold=0.5  InputSameDT=on
  Terminator : Terminator
  Unit Delay : UnitDelay  Orientation=left  SampleTime=-1
  y : Outport
  wires:
  Memory/1 -> Relational Operator/2
  Unit Delay/1 -> Sum/2
  Switch/1 -> Unit Delay/1
  Gain1/1 -> Switch/3
  Relational Operator/1 -> Switch/2
  Sum/1 -> Switch/1, Fcn/1
  Probe/1 -> Sum/1, Gain1/1
  u/1 -> Memory/1, Probe/1, Relational Operator/1
  Fcn/1 -> y/1
  Probe/2 -> Terminator/1

== system xpclib/Misc./To xPC Target /Subsystem ==
  In1 : Inport  LatchInput=off
  Enable : EnablePort
  S-Function : S-Function  FunctionName=dng2xpc  Parameters=paramid
  wires:
  In1/1 -> S-Function/1

== system xpclib/RS232/Asynchronous Mode/Receive  ==
  S-Function : S-Function  FunctionName=rs232_rec  Parameters=port,formatrec,numb,ts
  Out1 : Outport
  wires:
  S-Function/1 -> Out1/1

== system xpclib/RS232/Asynchronous Mode/Send  ==
  In1 : Inport  LatchInput=off
  S-Function : S-Function  FunctionName=rs232_send  Parameters=port,formatsend,wait,ts
  wires:
  In1/1 -> S-Function/1

== system xpclib/RS232/Diamond/Emerald-MM  ==
  Diamond Emerald-MM : Subsystem  PropExecContextAcrossSSBoundary=on
  Diamond Emerald-MM Serial : Subsystem  InitFcn=mdiamondemeraldmask(4,4);  TreatAsAtomicUnit=on  PropExecContextAcrossSSBoundary=on  mask(Emerald-MM RS232 Send Receive){group=Board Setup, port=1, irqnum=7, saddr1=0x240, baud1=115200, parity1=None, ndata1=8, nstop1=1, fifomode1=16 deep, rlevel1=half full, automode1=on, xmtfifosize1=1024, xmtdatatype1=8 bit uint null terminated, rcvfifosize1=1024, rcvmaxread1=1024, rcvminread1=1, rcvusedelim1=on, rcvdelim1=13, rcvdatatype1=count+16 bit uint, rcvsampletime1=-1, baud2=115200, parity2=None, ndata2=8, nstop2=1, fifomode2=16 deep, rlevel2=half full, automode2=on, xmtfifosize2=1024, xmtdatatype2=8 bit uint null terminated, rcvfifosize2=1024, rcvmaxread2=1024, rcvminread2=1, rcvusedelim2=on, rcvdelim2=13, rcvdatatype2=count+16 bit uint, rcvsampletime2=-1, baud3=115200, parity3=None, ndata3=8, nstop3=1, fifomode3=16 deep, rlevel3=half full, automode3=on, xmtfifosize3=1024, xmtdatatype3=8 bit uint null terminated, rcvfifosize3=1024, rcvmaxread3=1024, rcvminread3=1, rcvusedelim3=on, rcvdelim3=13, rcvdatatype3=count+16 bit uint, rcvsampletime3=-1, baud4=115200, parity4=None, ndata4=8, nstop4=1, fifomode4=16 deep, rlevel4=half full, automode4=on, xmtfifosize4=1024, xmtdatatype4=8 bit uint null terminated, rcvfifosize4=1024, rcvmaxread4=1024, rcvminread4=1, rcvusedelim4=on, rcvdelim4=13, rcvdatatype4=count+16 bit uint, rcvsampletime4=-1}
      mask prompts: group "Parameter group:"; port "Port to modify:"; irqnum "IRQ number:"; saddr1 "First port address:"; baud1 "Baud rate:"; parity1 "Parity:"; ndata1 "Data bits:"; nstop1 "Stop bits:"; fifomode1 "Hardware fifo size:"; rlevel1 "Receive fifo interrupt level:"; automode1 "Auto RTS/CTS:"; xmtfifosize1 "Transmit software fifo size:"; xmtdatatype1 "Transmit fifo data type:"; rcvfifosize1 "Receive software fifo size:"; rcvmaxread1 "Receive maximum read:"; rcvminread1 "Receive minimum read:"; rcvusedelim1 "Read to delimiter:"; rcvdelim1 "Delimiter:"; rcvdatatype1 "Receive data type:"; rcvsampletime1 "Receive SampleTime:"; baud2 "Baud rate:"; parity2 "Parity:"; ndata2 "Data bits:"; nstop2 "Stop bits:"; fifomode2 "Hardware fifo size:"; rlevel2 "Receive fifo interrupt level:"; automode2 "Auto RTS/CTS:"; xmtfifosize2 "Transmit software fifo size:"; xmtdatatype2 "Transmit fifo data type:"; rcvfifosize2 "Receive software fifo size:"; rcvmaxread2 "Receive maximum read:"; rcvminread2 "Receive minimum read:"; rcvusedelim2 "Read to delimiter:"; rcvdelim2 "Delimiter:"; rcvdatatype2 "Receive data type:"; rcvsampletime2 "Receive SampleTime:"; baud3 "Baud rate:"; parity3 "Parity:"; ndata3 "Data bits:"; nstop3 "Stop bits:"; fifomode3 "Hardware fifo size:"; rlevel3 "Receive fifo interrupt level:"; automode3 "Auto RTS/CTS:"; xmtfifosize3 "Transmit software fifo size:"; xmtdatatype3 "Transmit fifo data type:"; rcvfifosize3 "Receive software fifo size:"; rcvmaxread3 "Receive maximum read:"; rcvminread3 "Receive minimum read:"; rcvusedelim3 "Read to delimiter:"; rcvdelim3 "Delimiter:"; rcvdatatype3 "Receive data type:"; rcvsampletime3 "Receive SampleTime:"; baud4 "Baud rate:"; parity4 "Parity:"; ndata4 "Data bits:"; nstop4 "Stop bits:"; fifomode4 "Hardware fifo size:"; rlevel4 "Receive fifo interrupt level:"; automode4 "Auto RTS/CTS:"; xmtfifosize4 "Transmit software fifo size:"; xmtdatatype4 "Transmit fifo data type:"; rcvfifosize4 "Receive software fifo size:"; rcvmaxread4 "Receive maximum read:"; rcvminread4 "Receive minimum read:"; rcvusedelim4 "Read to delimiter:"; rcvdelim4 "Delimiter:"; rcvdatatype4 "Receive data type:"; rcvsampletime4 "Receive SampleTime:"
      mask help:
      | Diamond Emerald
      | RS232 Send Receive Subsystem
      mask init:
      | addr = mdiamondemeraldmask( 1, 4 );
      | baddr1 = addr{1};
      | baddr2 = addr{2};
      | baddr3 = addr{3};
      | baddr4 = addr{4};
      | istat = addr{5};
      | mdiamondemeraldmask( 3, 4 );
      mask Help: helpview(fullfile(docroot, 'mapfiles', 'xpc.map'), 'Baseboard_Serial_Subsystem')
      mask StyleString: popup(Board Setup|Basic Setup|Transmit Setup|Receive Setup),popup(1|2|3|4),edit,popup(0x3F8|0x3E8|0x380|0x240|0x100|0x120|0x140|0x160),popup(921600|460800|230400|115200|57600|38400|19200|9600|4800|2400|1200|600|300|110),popup(None|Even|Odd|Mark|Space),popup(5|6|7|8),popup(1|2),popup(64 deep|16 deep|1 deep),popup(1|quarter full|half full|almost full),checkbox,edit,popup(count+32 bit int|count+32 bit uint|count+16 bit int|count+16 bit uint|8 bit int null terminated|8 bit uint null terminated),edit,edit,edit,checkbox,edit,popup(count+32 bit int|count+32 bit uint|count+16 bit int|count+16 bit uint|8 bit int null terminated|8 bit uint null terminated),edit,popup(921600|460800|230400|115200|57600|38400|19200|9600|4800|2400|1200|600|300|110),popup(None|Even|Odd|Mark|Space),popup(5|6|7|8),popup(1|2),popup(64 deep|16 deep|1 deep),popup(1|quarter full|half full|almost full),checkbox,edit,popup(count+32 bit int|count+32 bit uint|count+16 bit int|count+16 bit uint|8 bit int null terminated|8 bit uint null terminated),edit,edit,edit,checkbox,edit,popup(count+32 bit int|count+32 bit uint|count+16 bit int|count+16 bit uint|8 bit int null terminated|8 bit uint null terminated),edit,popup(921600|460800|230400|115200|57600|38400|19200|9600|4800|2400|1200|600|300|110),popup(None|Even|Odd|Mark|Space),popup(5|6|7|8),popup(1|2),popup(64 deep|16 deep|1 deep),popup(1|quarter full|half full|almost full),checkbox,edit,popup(count+32 bit int|count+32 bit uint|count+16 bit int|count+16 bit uint|8 bit int null terminated|8 bit uint null terminated),edit,edit,edit,checkbox,edit,popup(count+32 bit int|count+32 bit uint|count+16 bit int|count+16 bit uint|8 bit int null terminated|8 bit uint null terminated),edit,popup(921600|460800|230400|115200|57600|38400|19200|9600|4800|2400|1200|600|300|110),popup(None|Even|Odd|Mark|Space),popup(5|6|7|8),popup(1|2),popup(64 deep|16 deep|1 deep),popup(1|quarter full|half full|almost full),checkbox,edit,popup(count+32 bit int|count+32 bit uint|count+16 bit int|count+16 bit uint|8 bit int null terminated|8 bit uint null terminated),edit,edit,edit,checkbox,edit,popup(count+32 bit int|count+32 bit uint|count+16 bit int|count+16 bit uint|8 bit int null terminated|8 bit uint null terminated),edit
      mask CallbackString:
      | mdiamondemeraldmask( 2, 4 );
      | |mdiamondemeraldmask( 2, 4 );||||||||||||||||||||||||||||||||||||||||||||||||||||||||||||||||||
      mask Display:
      | disp('Diamond\n\nEmerald\nRS232\nSend Receive');
      | port_label('input',1,'XMT1');
      | port_label('input',2,'XMT2');
      | port_label('input',3,'XMT3');
      | port_label('input',4,'XMT4');
      | port_label('output',1,'RCV1');
      | port_label('output',2,'RCV2');
      | port_label('output',3,'RCV3');
      | port_label('output',4,'RCV4');
  "Modem Control " : S-Function  InitFcn=mmodemcontrol(5);  FunctionName=modemcontrolemeraldmm  Parameters=addr, boardtype, rts, dtr, count  mask(Modem Control){port=1, rts=on, dtr=on, firstaddr=0x240}
      mask prompts: firstaddr "First port address:"
      mask help:
      | Diamond Emerald-MM
      | Modem Control
      mask init:
      | count = 0;
      | boardtype = 5;
      | [maskdisplay, count, addr] = mmodemcontrol( 2, rts, dtr, boardtype, port, firstaddr );
      | addr = hex2dec( addr(3:end) );
      | set_param( gcb, 'MaskDisplay', maskdisplay );
      mask Help: helpview(fullfile(docroot, 'mapfiles', 'xpc.map'), 'Emerald_MODEM_Control')
      mask StyleString: popup(1|2|3|4),checkbox,checkbox,popup(0x3F8|0x3E8|0x380|0x240|0x100|0x120|0x140)
      mask Display: disp('Diamond\nEmerald-MM\nModem Control');port_label('input',1,'RTS');port_label('input',2,'DTR');
  "Modem Status " : S-Function  FunctionName=modemstatusemeraldmm  Parameters=addr, boardtype, cts, dsr, ring, dcd, count, sampletime  mask(Modem Status){port=1, cts=on, dsr=on, ring=on, dcd=on, sampletime=-1, firstaddr=0x240}
      mask prompts: ring "RI:"; firstaddr "First port address:"
      mask help:
      | Diamond Emerald-MM
      | Modem Status
      mask init:
      | count = 0;
      | boardtype = 5;
      | [maskdisplay, count, addr] = mmodemstatus( 2, cts, dsr, ring, dcd, boardtype, port, firstaddr );
      | addr = hex2dec( addr(3:end) );
      | set_param( gcb, 'MaskDisplay', maskdisplay );
      mask Help: helpview(fullfile(docroot, 'mapfiles', 'xpc.map'), 'Emerald_MODEM_Status')
      mask StyleString: popup(1|2|3|4),checkbox,checkbox,checkbox,checkbox,edit,popup(0x3F8|0x3E8|0x380|0x240|0x100|0x120|0x140)
      mask Display: disp('Diamond\nEmerald-MM\nModem Status');port_label('output',1,'CTS');port_label('output',2,'DSR');port_label('output',3,'RI');port_label('output',4,'DCD');
